simulink model "SVM_3_lev_full_R2021a"  (R2021a)
settings: Solver=ode45  StartTime=0.0  StopTime=0.1  MaxStep=5e-6  RelTol=1e-3
settings Model: Creator=amogh  LastModifiedBy=amogh
settings DebuggingCC: UnconnectedInputMsg=none  UnconnectedOutputMsg=none  UnconnectedLineMsg=none
settings ModelReferenceCC: EnableRefExpFcnMdlSchedulingChecks=off
settings RTWCC: Description=Generic Real-Time Target  GPUComputeCapability=5.0  DLArmComputeVersion=20.02.1

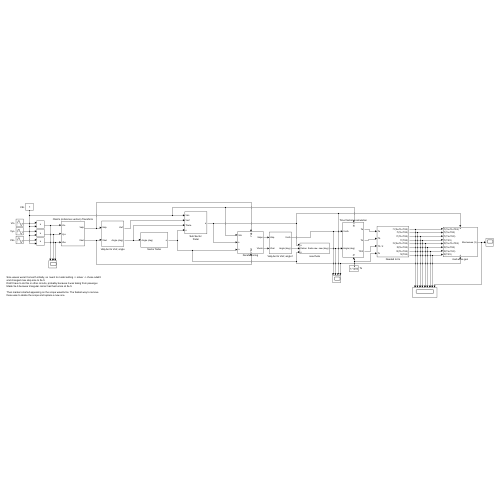
[thumbnail: Simulink's stored preview of the top-level diagram]
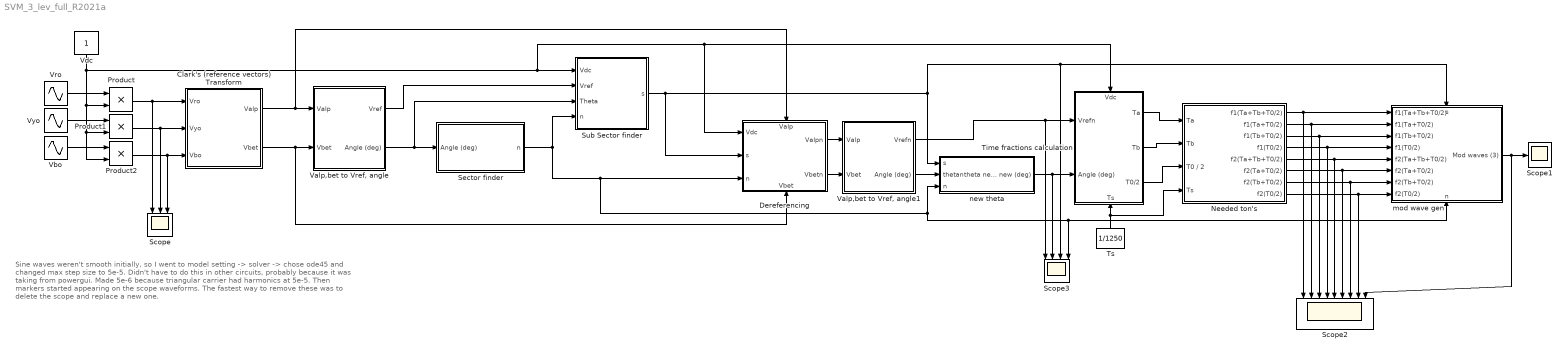
== system SVM_3_lev_full_R2021a ==
  note: Sine waves weren't smooth initially, so I went to model setting -> solver -> chose ode45 and changed max step size to 5e-5.
      | Didn't have to do this in other circuits, probably because it was taking from powergui.
      | Made 5e-6 because triangular carrier had harmonics at 5e-5.
      |
      | Then markers started appearing on the scope waveforms. The fastest way to remove these was to delete the scope and replace a new one.
  Clark's (reference vectors) Transform : Subsystem
  Dereferencing : Subsystem
      settings: PortSchema="{\"entries\":[{\"content\":{\"sides\":[{\"content\":{\"connectorIds\":[\"In1\",\"In2\",\"In3\"]},\"type\":\"ConnectorPlacement.EquallySpacedRectSide\",\"uuid\":\"ecd07562-dffd-4a2a-9a36-330545a18d82\"},{\"content\":{\"connectorIds\":[\"Out1\",\"Out2\"],\"side\":\"RIGHT\"},\"type\":\"ConnectorPlacement.EquallySpacedRectSide\",\"uuid\":\"ea8e31d3-a9b9-4759-a79b-beda552eeb92\"},{\"content\":{\"connectorIds\":[\"In4\"],\"side\":\"TOP\"},\"type\":\"ConnectorPlacement.EquallySpacedRectSide\",\"uuid\":\"419a6bdf-1295-4686-a05a-cf3461a06939\"},{\"content\":{\"connectorIds\":[\"In5\"],\"side\":\"BOTTOM\"},\"type\":\"ConnectorPlacement.EquallySpacedRectSide\",\"uuid\":\"ae539f20-9b7e-461f-b0b3-230075384a0b\"}]},\"type\":\"ConnectorPlacement.EquallySpacedConnector\",\"uuid\":\"6cf660ee-94cd-474a-b972-1e1c5d4c87d4\"}],\"packageUris\":[\"http://schema.mathworks.com/mf0/Connector/R2020b\"],\"version\":\"1.0\"}"
  Needed ton's : Subsystem
  Product : Product
  Product1 : Product
  Product2 : Product
  Scope : Scope  NumInputPorts=3
  Scope1 : Scope
  Scope2 : Scope  NumInputPorts=9
  Scope3 : Scope  NumInputPorts=4
  Sector finder : Subsystem
  Sub Sector finder : Subsystem
  Time fractions calculation : Subsystem
      settings: PortSchema="{\"entries\":[{\"content\":{\"sides\":[{\"content\":{\"connectorIds\":[\"In1\",\"In2\"]},\"type\":\"ConnectorPlacement.EquallySpacedRectSide\",\"uuid\":\"39dbe934-5c3a-4725-abbb-a0301a466b70\"},{\"content\":{\"connectorIds\":[\"Out1\",\"Out2\",\"Out3\"],\"side\":\"RIGHT\"},\"type\":\"ConnectorPlacement.EquallySpacedRectSide\",\"uuid\":\"4a451c39-d3ce-4daa-ad2d-b84a18627464\"},{\"content\":{\"connectorIds\":[\"In3\"],\"side\":\"TOP\"},\"type\":\"ConnectorPlacement.EquallySpacedRectSide\",\"uuid\":\"7f465595-a607-4b7f-b400-abaa5826d345\"},{\"content\":{\"connectorIds\":[\"In4\"],\"side\":\"BOTTOM\"},\"type\":\"ConnectorPlacement.EquallySpacedRectSide\",\"uuid\":\"0791232b-36d2-4a91-ab81-b8e525b336bd\"}]},\"type\":\"ConnectorPlacement.EquallySpacedConnector\",\"uuid\":\"bf18cf26-6ee3-4127-84f4-4a6b0242db08\"}],\"packageUris\":[\"http://schema.mathworks.com/mf0/Connector/R2020b\"],\"version\":\"1.0\"}"
  Ts : Constant  Value=1/1250
  "Valp,bet to Vref, angle" : Subsystem
  "Valp,bet to Vref, angle1" : Subsystem
  Vbo : Sin  Amplitude=1/(2)  Frequency=314.15926536  Phase=2*pi/3  SampleTime=0
  Vdc : Constant
  Vro : Sin  Amplitude=1/(2)  Frequency=314.15926536  SampleTime=0
  Vyo : Sin  Amplitude=1/(2)  Frequency=314.15926536  Phase=-2*pi/3  SampleTime=0
  mod wave gen : Subsystem
      settings: PortSchema="{\"entries\":[{\"content\":{\"sides\":[{\"content\":{\"connectorIds\":[\"In1\",\"In2\",\"In3\",\"In4\",\"In5\",\"In6\",\"In7\",\"In8\"]},\"type\":\"ConnectorPlacement.EquallySpacedRectSide\",\"uuid\":\"db72baa2-f5a7-4ee9-9029-042c80451c67\"},{\"content\":{\"connectorIds\":[\"Out1\"],\"side\":\"RIGHT\"},\"type\":\"ConnectorPlacement.EquallySpacedRectSide\",\"uuid\":\"6ae855a2-30a9-4ffd-942e-d2978ed01332\"},{\"content\":{\"connectorIds\":[\"In9\"],\"side\":\"TOP\"},\"type\":\"ConnectorPlacement.EquallySpacedRectSide\",\"uuid\":\"4df407e7-466e-4838-b593-b1b4063e48fa\"},{\"content\":{\"connectorIds\":[\"In10\"],\"side\":\"BOTTOM\"},\"type\":\"ConnectorPlacement.EquallySpacedRectSide\",\"uuid\":\"76c4a454-b21e-401b-80ad-65be32248efa\"}]},\"type\":\"ConnectorPlacement.EquallySpacedConnector\",\"uuid\":\"31301616-82a2-448c-a283-a7a359799af9\"}],\"packageUris\":[\"http://schema.mathworks.com/mf0/Connector/R2020b\"],\"version\":\"1.0\"}"
  new theta : Subsystem
  wires:
  Vbo/1 -> Product2/1
  Product1/1 -> Scope/2, Clark's (reference vectors) Transform/2(Vyo)
  Vro/1 -> Product/1
  Product/1 -> Clark's (reference vectors) Transform/1(Vro), Scope/1
  Vdc/1 -> Product/2, Product1/2, Product2/2, Time fractions calculation/3(Vdc), Dereferencing/1(Vdc), Sub Sector finder/1(Vdc)
  "Valp,bet to Vref, angle"/2(Angle (deg)) -> Sub Sector finder/3(Theta), Sector finder/1(Angle (deg))
  Vyo/1 -> Product1/1
  Clark's (reference vectors) Transform/1(Valp) -> "Valp,bet to Vref, angle"/1(Valp), Dereferencing/4(Valp)
  Clark's (reference vectors) Transform/2(Vbet) -> "Valp,bet to Vref, angle"/2(Vbet), Dereferencing/5(Vbet)
  Product2/1 -> Scope/3, Clark's (reference vectors) Transform/3(Vbo)
  "Valp,bet to Vref, angle"/1(Vref) -> Sub Sector finder/2(Vref)
  Sector finder/1(n) -> Scope3/4, mod wave gen/10(n), new theta/3(n), Dereferencing/3(n), Sub Sector finder/4(n)
  Sub Sector finder/1(s) -> Dereferencing/2(s), mod wave gen/9(s), Scope3/3, new theta/1(s)
  Dereferencing/2(Vbetn) -> "Valp,bet to Vref, angle1"/2(Vbet)
  Dereferencing/1(Valpn) -> "Valp,bet to Vref, angle1"/1(Valp)
  "Valp,bet to Vref, angle1"/2(Angle (deg)) -> new theta/2(thetan)
  new theta/1(theta new new (deg)) -> Time fractions calculation/2(Angle (deg)), Scope3/2
  Ts/1 -> Needed ton's/4(Ts), Time fractions calculation/4(Ts)
  "Valp,bet to Vref, angle1"/1(Vrefn) -> Time fractions calculation/1(Vrefn), Scope3/1
  Time fractions calculation/2(Tb) -> Needed ton's/2(Tb)
  Time fractions calculation/1(Ta) -> Needed ton's/1(Ta)
  Time fractions calculation/3(T0/2) -> Needed ton's/3(T0 / 2)
  Needed ton's/1(f1(Ta+Tb+T0/2)) -> Scope2/1, mod wave gen/1(f1(Ta+Tb+T0/2))
  Needed ton's/2(f1(Ta+T0/2)) -> Scope2/2, mod wave gen/2(f1(Ta+T0/2))
  Needed ton's/3(f1(Tb+T0/2)) -> Scope2/3, mod wave gen/3(f1(Tb+T0/2))
  Needed ton's/4(f1(T0/2)) -> Scope2/4, mod wave gen/4(f1(T0/2))
  Needed ton's/5(f2(Ta+Tb+T0/2)) -> mod wave gen/5(f2(Ta+Tb+T0/2)), Scope2/5
  Needed ton's/6(f2(Ta+T0/2)) -> mod wave gen/6(f2(Ta+T0/2)), Scope2/6
  Needed ton's/7(f2(Tb+T0/2)) -> mod wave gen/7(f2(Tb+T0/2)), Scope2/7
  Needed ton's/8(f2(T0/2)) -> mod wave gen/8(f2(T0/2)), Scope2/8
  mod wave gen/1(Mod waves (3)) -> Scope2/9, Scope1/1

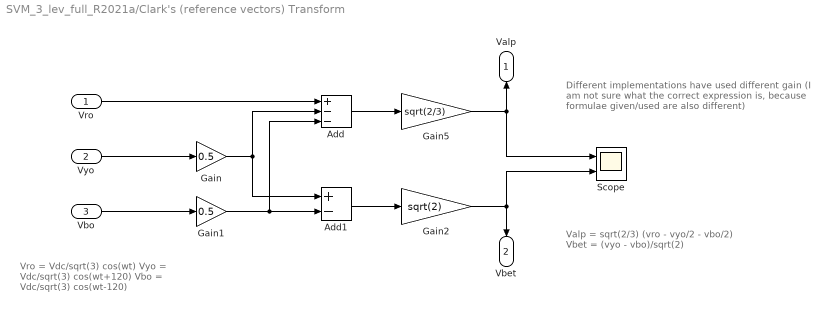
== system SVM_3_lev_full_R2021a/Clark's (reference vectors) Transform ==
  note: Different implementations have used different gain
      | (I am not sure what the correct expression is, because formulae given/used are also different)
  note: Vro = Vdc/sqrt(3) cos(wt)
      | Vyo = Vdc/sqrt(3) cos(wt+120)
      | Vbo = Vdc/sqrt(3) cos(wt-120)
  note: Valp = sqrt(2/3) (vro - vyo/2 - vbo/2)
      | Vbet = (vyo - vbo)/sqrt(2)
  Vro : Inport
  Vyo : Inport  Port=2
  Vbo : Inport  Port=3
  Add : Sum  Inputs=+--
  Add1 : Sum  Inputs=+-
  Gain : Gain  Gain=0.5
  Gain1 : Gain  Gain=0.5
  Gain2 : Gain  Gain=sqrt(2)
  Gain5 : Gain  Gain=sqrt(2/3)
  Scope : Scope  NumInputPorts=2
  Valp : Outport
  Vbet : Outport  Port=2
  wires:
  Vro/1 -> Add/1
  Gain1/1 -> Add1/2, Add/3
  Gain/1 -> Add/2, Add1/1
  Vbo/1 -> Gain1/1
  Vyo/1 -> Gain/1
  Add/1 -> Gain5/1
  Gain5/1 -> Scope/1, Valp/1
  Add1/1 -> Gain2/1
  Gain2/1 -> Scope/2, Vbet/1

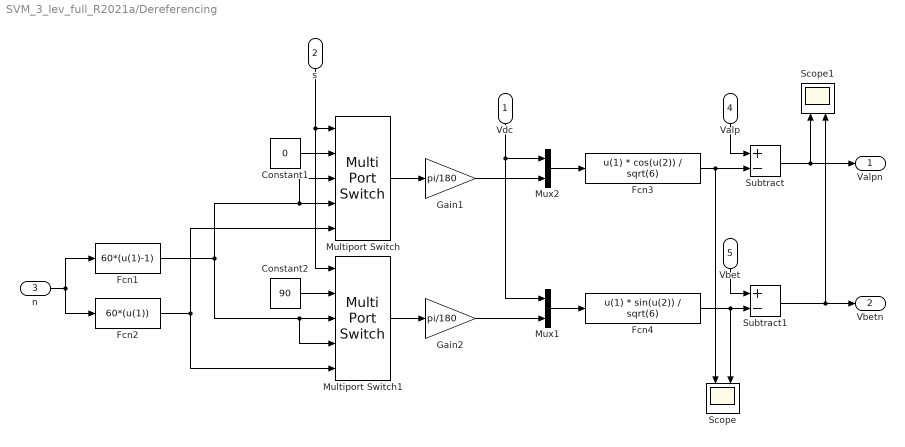
== system SVM_3_lev_full_R2021a/Dereferencing ==
  Vdc : Inport
  s : Inport  Port=2
  n : Inport  Port=3
  Valp : Inport  Port=4
  Vbet : Inport  Port=5
  Constant1 : Constant  Value=0
  Constant2 : Constant  Value=90
  Fcn1 : Fcn  Expr=60*(u(1)-1)
  Fcn2 : Fcn  Expr=60*(u(1))
  Fcn3 : Fcn  Expr=u(1) * cos(u(2)) / sqrt(6)
  Fcn4 : Fcn  Expr=u(1) * sin(u(2)) / sqrt(6)
  Gain1 : Gain  Gain=pi/180
  Gain2 : Gain  Gain=pi/180
  Multiport Switch : MultiPortSwitch  Inputs=4
  Multiport Switch1 : MultiPortSwitch  Inputs=4
  Mux1 : Mux  Inputs=2
  Mux2 : Mux  Inputs=2
  Scope : Scope  NumInputPorts=2
  Scope1 : Scope  NumInputPorts=2
  Subtract : Sum  Inputs=+-
  Subtract1 : Sum  Inputs=+-
  Valpn : Outport
  Vbetn : Outport  Port=2
  wires:
  s/1 -> Multiport Switch1/1, Multiport Switch/1
  Fcn2/1 -> Multiport Switch/5, Multiport Switch1/5
  Mux1/1 -> Fcn4/1
  Vbet/1 -> Subtract1/1
  Valp/1 -> Subtract/1
  Constant1/1 -> Multiport Switch/2
  Multiport Switch/1 -> Gain1/1
  Fcn1/1 -> Multiport Switch/3, Multiport Switch/4, Multiport Switch1/4, Multiport Switch1/3
  n/1 -> Fcn1/1, Fcn2/1
  Mux2/1 -> Fcn3/1
  Gain2/1 -> Mux1/2
  Fcn3/1 -> Subtract/2, Scope/1
  Fcn4/1 -> Scope/2, Subtract1/2
  Vdc/1 -> Mux1/1, Mux2/1
  Multiport Switch1/1 -> Gain2/1
  Gain1/1 -> Mux2/2
  Constant2/1 -> Multiport Switch1/2
  Subtract1/1 -> Vbetn/1, Scope1/2
  Subtract/1 -> Valpn/1, Scope1/1

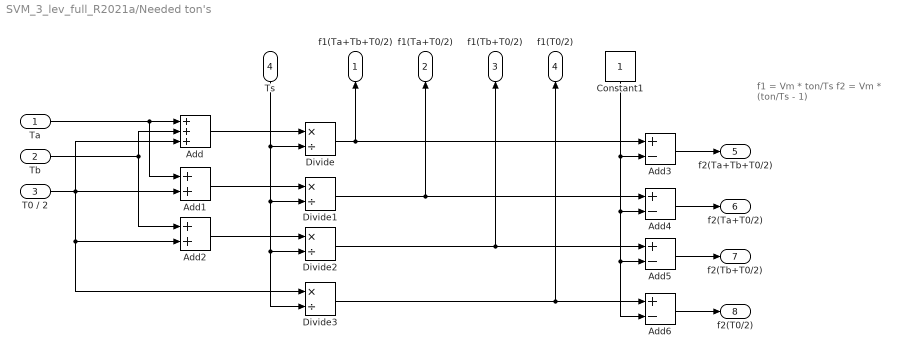
== system SVM_3_lev_full_R2021a/Needed ton's ==
  note: f1 = Vm * ton/Ts
      | f2 = Vm * (ton/Ts - 1)
  Ta : Inport
  Tb : Inport  Port=2
  T0 / 2 : Inport  Port=3
  Ts : Inport  Port=4
  Add : Sum  Inputs=+++
  Add1 : Sum
  Add2 : Sum
  Add{3..6} (4 alike) : Sum  Inputs=+-
  Constant1 : Constant
  Divide{,1..3} (4 alike) : Product  Inputs=*/
  f1(Ta+Tb+T0/2) : Outport
  f1(Ta+T0/2) : Outport  Port=2
  f1(Tb+T0/2) : Outport  Port=3
  f1(T0/2) : Outport  Port=4
  f2(Ta+Tb+T0/2) : Outport  Port=5
  f2(Ta+T0/2) : Outport  Port=6
  f2(Tb+T0/2) : Outport  Port=7
  f2(T0/2) : Outport  Port=8
  wires:
  T0 / 2/1 -> Add1/2, Add/3, Divide3/1, Add2/2
  Tb/1 -> Add/2, Add2/1
  Ta/1 -> Add1/1, Add/1
  Add2/1 -> Divide2/1
  Add1/1 -> Divide1/1
  Add/1 -> Divide/1
  Ts/1 -> Divide3/2, Divide2/2, Divide1/2, Divide/2
  Divide/1 -> f1(Ta+Tb+T0/2)/1, Add3/1
  Divide1/1 -> Add4/1, f1(Ta+T0/2)/1
  Divide2/1 -> f1(Tb+T0/2)/1, Add5/1
  Add4/1 -> f2(Ta+T0/2)/1
  Add5/1 -> f2(Tb+T0/2)/1
  Constant1/1 -> Add3/2, Add6/2, Add5/2, Add4/2
  Divide3/1 -> f1(T0/2)/1, Add6/1
  Add6/1 -> f2(T0/2)/1
  Add3/1 -> f2(Ta+Tb+T0/2)/1

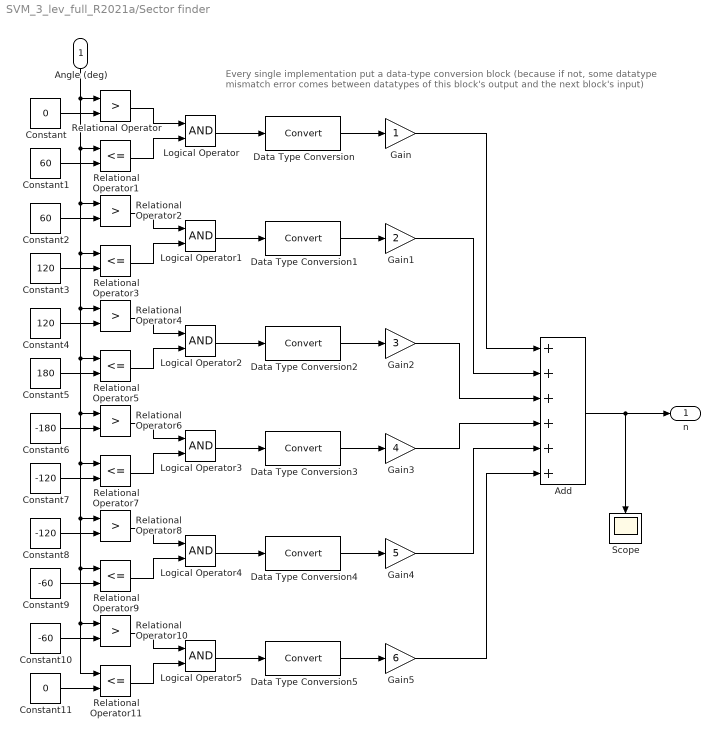
== system SVM_3_lev_full_R2021a/Sector finder ==
  note: Every single implementation put a data-type conversion block (because if not, some datatype mismatch error comes between datatypes of this block's output and the next block's input)
  Angle (deg) : Inport
  Add : Sum  Inputs=++++++
  Constant : Constant  Value=0
  Constant1 : Constant  Value=60
  Constant10 : Constant  Value=-60
  Constant11 : Constant  Value=0
  Constant2 : Constant  Value=60
  Constant3 : Constant  Value=120
  Constant4 : Constant  Value=120
  Constant5 : Constant  Value=180
  Constant6 : Constant  Value=-180
  Constant7 : Constant  Value=-120
  Constant8 : Constant  Value=-120
  Constant9 : Constant  Value=-60
  Data Type Conversion{,1..5} (6 alike) : DataTypeConversion
  Gain : Gain
  Gain1 : Gain  Gain=2
  Gain2 : Gain  Gain=3
  Gain3 : Gain  Gain=4
  Gain4 : Gain  Gain=5
  Gain5 : Gain  Gain=6
  Logical Operator{,1..5} (6 alike) : Logic  AllPortsSameDT=off  OutDataTypeStr=boolean
  Relational Operator{,2,4,6,8,10} (6 alike) : RelationalOperator  Operator=>  OutDataTypeStr=boolean  RndMeth=Simplest
  Relational Operator{1,3,5,7,9,11} (6 alike) : RelationalOperator  Operator=<=  OutDataTypeStr=boolean  RndMeth=Simplest
  Scope : Scope
  n : Outport
  wires:
  Constant11/1 -> Relational Operator11/2
  Gain3/1 -> Add/4
  Constant10/1 -> Relational Operator10/2
  Constant/1 -> Relational Operator/2
  Angle (deg)/1 -> Relational Operator11/1, Relational Operator10/1, Relational Operator9/1, Relational Operator8/1, Relational Operator7/1, Relational Operator6/1, Relational Operator5/1, Relational Operator4/1, Relational Operator3/1, Relational Operator2/1, Relational Operator1/1, Relational Operator/1
  Gain5/1 -> Add/6
  Constant7/1 -> Relational Operator7/2
  Relational Operator10/1 -> Logical Operator5/1
  Constant9/1 -> Relational Operator9/2
  Relational Operator11/1 -> Logical Operator5/2
  Gain1/1 -> Add/2
  Relational Operator8/1 -> Logical Operator4/1
  Constant8/1 -> Relational Operator8/2
  Relational Operator7/1 -> Logical Operator3/2
  Constant3/1 -> Relational Operator3/2
  Relational Operator2/1 -> Logical Operator1/1
  Constant2/1 -> Relational Operator2/2
  Relational Operator/1 -> Logical Operator/1
  Relational Operator3/1 -> Logical Operator1/2
  Gain4/1 -> Add/5
  Constant6/1 -> Relational Operator6/2
  Relational Operator5/1 -> Logical Operator2/2
  Relational Operator6/1 -> Logical Operator3/1
  Constant5/1 -> Relational Operator5/2
  Constant4/1 -> Relational Operator4/2
  Relational Operator4/1 -> Logical Operator2/1
  Constant1/1 -> Relational Operator1/2
  Relational Operator9/1 -> Logical Operator4/2
  Relational Operator1/1 -> Logical Operator/2
  Add/1 -> Scope/1, n/1
  Gain/1 -> Add/1
  Gain2/1 -> Add/3
  Data Type Conversion/1 -> Gain/1
  Logical Operator/1 -> Data Type Conversion/1
  Logical Operator1/1 -> Data Type Conversion1/1
  Data Type Conversion1/1 -> Gain1/1
  Logical Operator5/1 -> Data Type Conversion5/1
  Data Type Conversion5/1 -> Gain5/1
  Logical Operator4/1 -> Data Type Conversion4/1
  Data Type Conversion4/1 -> Gain4/1
  Logical Operator2/1 -> Data Type Conversion2/1
  Data Type Conversion2/1 -> Gain2/1
  Logical Operator3/1 -> Data Type Conversion3/1
  Data Type Conversion3/1 -> Gain3/1

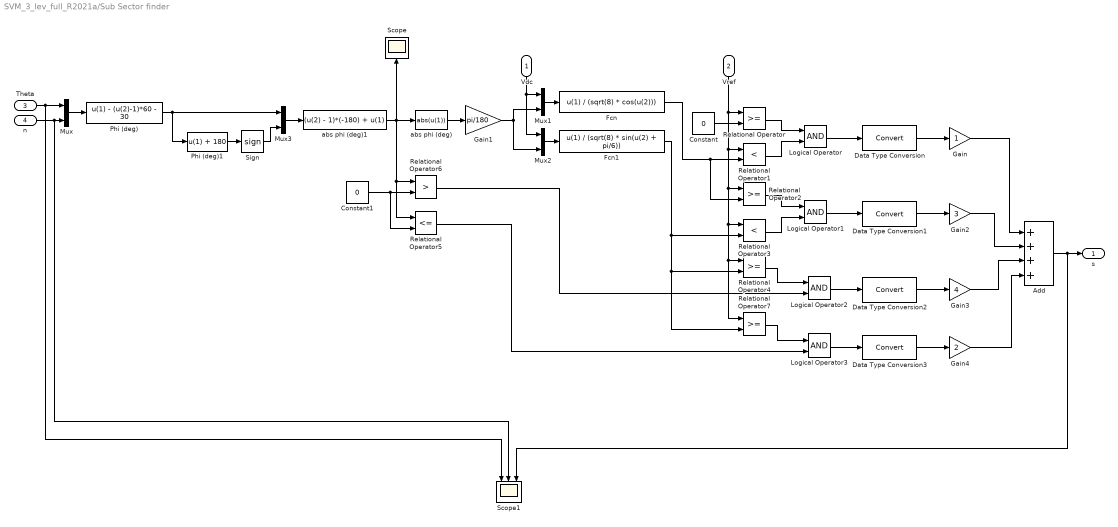
== system SVM_3_lev_full_R2021a/Sub Sector finder ==
  Vdc : Inport
  Vref : Inport  Port=2
  Theta : Inport  Port=3
  n : Inport  Port=4
  Add : Sum  Inputs=++++
  Constant : Constant  Value=0
  Constant1 : Constant  Value=0
  Data Type Conversion{,1..3} (4 alike) : DataTypeConversion
  Fcn : Fcn  Expr=u(1) / (sqrt(8) * cos(u(2)))
  Fcn1 : Fcn  Expr=u(1) / (sqrt(8) * sin(u(2) + pi/6))
  Gain : Gain
  Gain1 : Gain  Gain=pi/180
  Gain2 : Gain  Gain=3
  Gain3 : Gain  Gain=4
  Gain4 : Gain  Gain=2
  Logical Operator{,1..3} (4 alike) : Logic  AllPortsSameDT=off  OutDataTypeStr=boolean
  Mux{,1..3} (4 alike) : Mux  Inputs=2
  Phi (deg) : Fcn  Expr=u(1) - (u(2)-1)*60 - 30
  Phi (deg)1 : Fcn  Expr=u(1) + 180
  Relational Operator{,2,4,7} (4 alike) : RelationalOperator  OutDataTypeStr=boolean  RndMeth=Simplest
  Relational Operator1 : RelationalOperator  Operator=<  OutDataTypeStr=boolean  RndMeth=Simplest
  Relational Operator3 : RelationalOperator  Operator=<  OutDataTypeStr=boolean  RndMeth=Simplest
  Relational Operator5 : RelationalOperator  Operator=<=  OutDataTypeStr=boolean  RndMeth=Simplest
  Relational Operator6 : RelationalOperator  Operator=>  OutDataTypeStr=boolean  RndMeth=Simplest
  Scope : Scope
  Scope1 : Scope  NumInputPorts=3
  Sign : Signum  ZeroCross=off
  abs phi (deg) : Fcn  Expr=abs(u(1))
  abs phi (deg)1 : Fcn  Expr=(u(2) - 1)*(-180) + u(1)
  s : Outport
  wires:
  Mux1/1 -> Fcn/1
  Fcn/1 -> Relational Operator2/2, Relational Operator1/2
  Relational Operator6/1 -> Logical Operator2/2
  Relational Operator4/1 -> Logical Operator2/1
  Logical Operator3/1 -> Data Type Conversion3/1
  Fcn1/1 -> Relational Operator7/2, Relational Operator4/2, Relational Operator3/2
  Relational Operator3/1 -> Logical Operator1/2
  Data Type Conversion1/1 -> Gain2/1
  Constant1/1 -> Relational Operator5/2, Relational Operator6/2
  Vref/1 -> Relational Operator2/1, Relational Operator7/1, Relational Operator4/1, Relational Operator3/1, Relational Operator1/1, Relational Operator/1
  Mux/1 -> Phi (deg)/1
  Logical Operator1/1 -> Data Type Conversion1/1
  Gain3/1 -> Add/3
  Data Type Conversion/1 -> Gain/1
  Relational Operator2/1 -> Logical Operator1/1
  Gain/1 -> Add/1
  Theta/1 -> Mux/1, Scope1/1
  Relational Operator/1 -> Logical Operator/1
  Mux2/1 -> Fcn1/1
  Relational Operator1/1 -> Logical Operator/2
  n/1 -> Scope1/2, Mux/2
  Constant/1 -> Relational Operator/2
  Logical Operator/1 -> Data Type Conversion/1
  Gain4/1 -> Add/4
  Gain1/1 -> Mux1/2, Mux2/2
  Relational Operator5/1 -> Logical Operator3/2
  Gain2/1 -> Add/2
  Data Type Conversion2/1 -> Gain3/1
  Add/1 -> Scope1/3, s/1
  Vdc/1 -> Mux2/1, Mux1/1
  abs phi (deg)/1 -> Gain1/1
  Relational Operator7/1 -> Logical Operator3/1
  Data Type Conversion3/1 -> Gain4/1
  Logical Operator2/1 -> Data Type Conversion2/1
  abs phi (deg)1/1 -> abs phi (deg)/1, Relational Operator6/1, Relational Operator5/1, Scope/1
  Phi (deg)/1 -> Mux3/1, Phi (deg)1/1
  Mux3/1 -> abs phi (deg)1/1
  Sign/1 -> Mux3/2
  Phi (deg)1/1 -> Sign/1

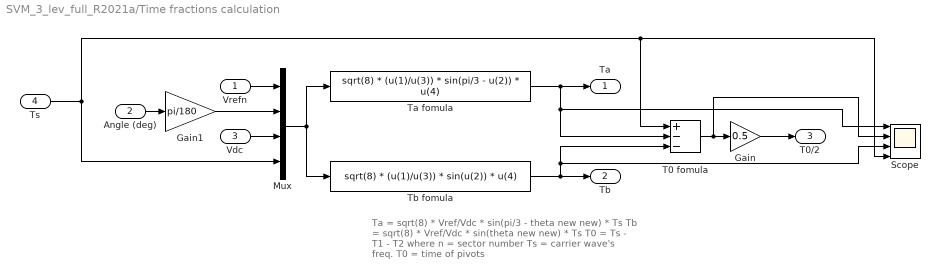
== system SVM_3_lev_full_R2021a/Time fractions calculation ==
  note: Ta = sqrt(8) * Vref/Vdc * sin(pi/3 - theta new new) * Ts
      | Tb = sqrt(8) * Vref/Vdc * sin(theta new new) * Ts
      | T0 = Ts - T1 - T2
      |
      | where 	n = sector number
      | 		Ts = carrier wave's freq.
      | 		T0 = time of pivots
  Vrefn : Inport
  Angle (deg) : Inport  Port=2
  Vdc : Inport  Port=3
  Ts : Inport  Port=4
  Gain : Gain  Gain=0.5
  Gain1 : Gain  Gain=pi/180
  Mux : Mux
  Scope : Scope  NumInputPorts=4
  T0 fomula : Sum  Inputs=+--
  Ta fomula : Fcn  Expr=sqrt(8) * (u(1)/u(3)) * sin(pi/3 - u(2)) * u(4)
  Tb fomula : Fcn  Expr=sqrt(8) * (u(1)/u(3)) * sin(u(2)) * u(4)
  Ta : Outport
  Tb : Outport  Port=2
  T0/2 : Outport  Port=3
  wires:
  Mux/1 -> Tb fomula/1, Ta fomula/1
  Tb fomula/1 -> Scope/3, T0 fomula/3, Tb/1
  Ta fomula/1 -> T0 fomula/2, Scope/1, Ta/1
  Ts/1 -> Mux/4, T0 fomula/1, Scope/4
  T0 fomula/1 -> Scope/2, Gain/1
  Gain/1 -> T0/2/1
  Angle (deg)/1 -> Gain1/1
  Vdc/1 -> Mux/3
  Gain1/1 -> Mux/2
  Vrefn/1 -> Mux/1

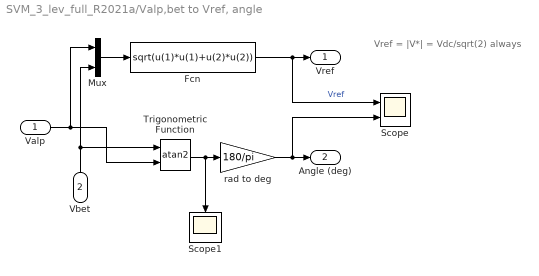
== system SVM_3_lev_full_R2021a/Valp,bet to Vref, angle ==
  note: Vref = |V*| = Vdc/sqrt(2) always
  Valp : Inport
  Vbet : Inport  Port=2
  Fcn : Fcn  Expr=sqrt(u(1)*u(1)+u(2)*u(2))
  Mux : Mux  Inputs=2
  Scope : Scope  NumInputPorts=2
  Scope1 : Scope
  Trigonometric Function : Trigonometry  Operator=atan2
  rad to deg : Gain  Gain=180/pi
  Vref : Outport
  Angle (deg) : Outport  Port=2
  wires:
  Valp/1 -> Mux/1, Trigonometric Function/2
  rad to deg/1 -> Scope/2, Angle (deg)/1
  Mux/1 -> Fcn/1
  Vbet/1 -> Trigonometric Function/1, Mux/2
  Fcn/1 -> Vref/1, Scope/1  "Vref"
  Trigonometric Function/1 -> Scope1/1, rad to deg/1

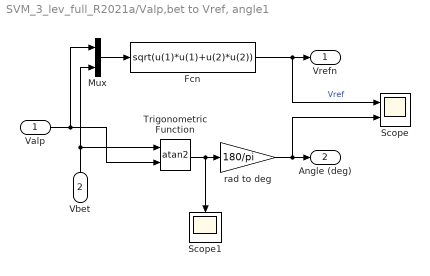
== system SVM_3_lev_full_R2021a/Valp,bet to Vref, angle1 ==
  Valp : Inport
  Vbet : Inport  Port=2
  Fcn : Fcn  Expr=sqrt(u(1)*u(1)+u(2)*u(2))
  Mux : Mux  Inputs=2
  Scope : Scope  NumInputPorts=2
  Scope1 : Scope
  Trigonometric Function : Trigonometry  Operator=atan2
  rad to deg : Gain  Gain=180/pi
  Vrefn : Outport
  Angle (deg) : Outport  Port=2
  wires:
  Valp/1 -> Mux/1, Trigonometric Function/2
  rad to deg/1 -> Scope/2, Angle (deg)/1
  Mux/1 -> Fcn/1
  Vbet/1 -> Trigonometric Function/1, Mux/2
  Fcn/1 -> Vrefn/1, Scope/1  "Vref"
  Trigonometric Function/1 -> Scope1/1, rad to deg/1

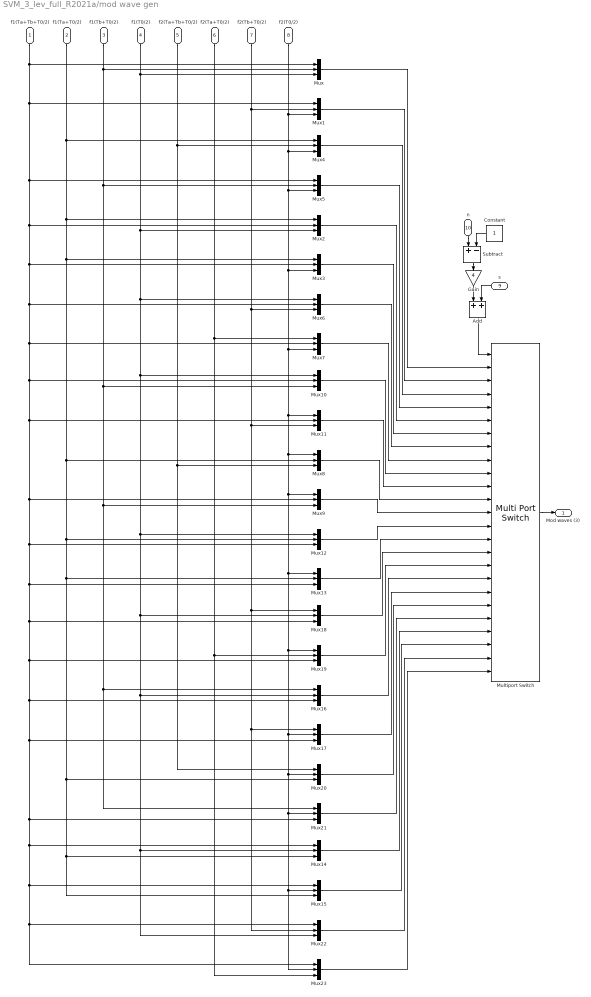
== system SVM_3_lev_full_R2021a/mod wave gen ==
  f1(Ta+Tb+T0/2) : Inport
  f1(Ta+T0/2) : Inport  Port=2
  f1(Tb+T0/2) : Inport  Port=3
  f1(T0/2) : Inport  Port=4
  f2(Ta+Tb+T0/2) : Inport  Port=5
  f2(Ta+T0/2) : Inport  Port=6
  f2(Tb+T0/2) : Inport  Port=7
  f2(T0/2) : Inport  Port=8
  s : Inport  Port=9
  n : Inport  Port=10
  Add : Sum
  Constant : Constant
  Gain : Gain  Gain=4
  Multiport Switch : MultiPortSwitch  Inputs=24
  Mux{,1..23} (24 alike) : Mux  Inputs=3
  Subtract : Sum  Inputs=+-
  Mod waves (3) : Outport
  wires:
  Mux1/1 -> Multiport Switch/3
  Multiport Switch/1 -> Mod waves (3)/1
  Mux5/1 -> Multiport Switch/5
  Mux3/1 -> Multiport Switch/7
  Mux4/1 -> Multiport Switch/4
  Mux2/1 -> Multiport Switch/6
  Mux/1 -> Multiport Switch/2
  Mux6/1 -> Multiport Switch/8
  Mux7/1 -> Multiport Switch/9
  Mux10/1 -> Multiport Switch/10
  Mux11/1 -> Multiport Switch/11
  Mux8/1 -> Multiport Switch/12
  Mux9/1 -> Multiport Switch/13
  Gain/1 -> Add/1
  s/1 -> Add/2
  Add/1 -> Multiport Switch/1
  Subtract/1 -> Gain/1
  n/1 -> Subtract/1
  Constant/1 -> Subtract/2
  Mux12/1 -> Multiport Switch/14
  Mux13/1 -> Multiport Switch/15
  Mux18/1 -> Multiport Switch/16
  Mux19/1 -> Multiport Switch/17
  Mux16/1 -> Multiport Switch/18
  Mux17/1 -> Multiport Switch/19
  Mux20/1 -> Multiport Switch/20
  Mux21/1 -> Multiport Switch/21
  Mux14/1 -> Multiport Switch/22
  Mux15/1 -> Multiport Switch/23
  Mux22/1 -> Multiport Switch/24
  Mux23/1 -> Multiport Switch/25
  f1(Ta+Tb+T0/2)/1 -> Mux/1, Mux1/1, Mux5/1, Mux2/2, Mux3/2, Mux6/2, Mux7/2, Mux10/2, Mux11/2, Mux9/2, Mux12/3, Mux13/3, Mux18/3, Mux19/3, Mux16/3, Mux17/3, Mux21/3, Mux14/1, Mux15/1, Mux22/1, Mux23/1
  f2(T0/2)/1 -> Mux1/3, Mux4/3, Mux5/3, Mux3/3, Mux7/3, Mux11/1, Mux8/1, Mux9/1, Mux13/1, Mux19/1, Mux17/2, Mux20/2, Mux21/2, Mux15/2, Mux23/2
  f2(Ta+T0/2)/1 -> Mux7/1, Mux19/2, Mux23/3
  f1(T0/2)/1 -> Mux/3, Mux2/3, Mux6/1, Mux10/1, Mux12/1, Mux18/2, Mux16/2, Mux14/2, Mux22/3
  f2(Tb+T0/2)/1 -> Mux1/2, Mux6/3, Mux11/3, Mux18/1, Mux17/1, Mux22/2
  f1(Ta+T0/2)/1 -> Mux4/1, Mux2/1, Mux3/1, Mux8/2, Mux12/2, Mux13/2, Mux20/3, Mux14/3, Mux15/3
  f1(Tb+T0/2)/1 -> Mux/2, Mux5/2, Mux10/3, Mux9/3, Mux16/1, Mux21/1
  f2(Ta+Tb+T0/2)/1 -> Mux8/3, Mux20/1, Mux4/2

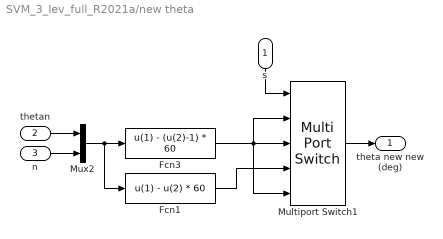
== system SVM_3_lev_full_R2021a/new theta ==
  s : Inport
  thetan : Inport  Port=2
  n : Inport  Port=3
  Fcn1 : Fcn  Expr=u(1) - u(2) * 60
  Fcn3 : Fcn  Expr=u(1) - (u(2)-1) * 60
  Multiport Switch1 : MultiPortSwitch  Inputs=4
  Mux2 : Mux  Inputs=2
  theta new new (deg) : Outport
  wires:
  Fcn1/1 -> Multiport Switch1/4
  Mux2/1 -> Fcn1/1, Fcn3/1
  thetan/1 -> Mux2/1
  Fcn3/1 -> Multiport Switch1/5, Multiport Switch1/3, Multiport Switch1/2
  s/1 -> Multiport Switch1/1
  n/1 -> Mux2/2
  Multiport Switch1/1 -> theta new new (deg)/1
